simulink model "ACCLogic_Test_Template"  (R2022b)
settings: Solver=FixedStepAuto  StartTime=0.0  StopTime=35  RelTol=1e-3  EnableMultiTasking=on
InitFcn:
  | ACCLogic_TestCase1
StopFcn:
  | ACCLogic_Plot
values from neighbouring files (symbols this model uses):
  Car1_start_s = 140    [ACCLogic_TestCase1.m]    (also in ACCLogic_TestCase2.m = 30)
  Car1_us = 0    [ACCLogic_TestCase1.m]    (also in ACCLogic_TestCase2.m)
  Car2_start_s = 42    [ACCLogic_TestCase1.m]    (also in ACCLogic_TestCase2.m = 47)
  Car2_us = 1.25    [ACCLogic_TestCase1.m]    (also in ACCLogic_TestCase2.m = 1)
  Car3_start_s = 25    [ACCLogic_TestCase1.m]    (also in ACCLogic_TestCase2.m)
  Car3_us = 0.25    [ACCLogic_TestCase1.m]    (also in ACCLogic_TestCase2.m)
  Car4_start_s = 95    [ACCLogic_TestCase1.m]    (also in ACCLogic_TestCase2.m = 35)
  Car4_us = 0.5    [ACCLogic_TestCase1.m]    (also in ACCLogic_TestCase2.m)
  Car5_start_s = 141    [ACCLogic_TestCase1.m]    (also in ACCLogic_TestCase2.m = 75)
  Car5_us = 0    [ACCLogic_TestCase1.m]    (also in ACCLogic_TestCase2.m)
  Car6_start_s = 142    [ACCLogic_TestCase1.m]    (also in ACCLogic_TestCase2.m = 30)
  Car6_us = 0    [ACCLogic_TestCase1.m]    (also in ACCLogic_TestCase2.m = 0.2)
  ManEnt1 = 10    [ACCLogic_TestCase1.m]    (also in ACCLogic_TestCase2.m)
  ManEnt2 = 15    [ACCLogic_TestCase1.m]    (also in ACCLogic_TestCase2.m)
  ManEnt3 = 20    [ACCLogic_TestCase1.m]    (also in ACCLogic_TestCase2.m)
  ManEnt4 = 25    [ACCLogic_TestCase1.m]    (also in ACCLogic_TestCase2.m)
  MyCarMan_us = 6    [ACCLogic_TestCase1.m]    (also in ACCLogic_TestCase2.m)
  MyCarVel_us = 3    [ACCLogic_TestCase1.m]    (also in ACCLogic_TestCase2.m)
  TIMESTEP = 0.01    [ACCLogic_TestCase1.m]    (also in ACCLogic_TestCase2.m)
libraries: simulink x6
settings Model: Creator=raoulkumar  LastModifiedBy=ryshaw
settings SolverCC: AlgebraicLoopSolver=TrustRegion
settings DataIOCC: SaveFormat=Array  ReturnWorkspaceOutputs=off
settings OptimizationCC: LifeSpan=inf
settings DebuggingCC: UnconnectedInputMsg=warning  UnconnectedOutputMsg=warning  UnconnectedLineMsg=warning  AllowSymbolicDim=off  SFUnexpectedBacktrackingDiag=warning  SFNoUnconditionalDefaultTransitionDiag=warning  SFExecutionAtInitializationDiag=none  SFMachineParentedDataDiag=warning  ArithmeticOperatorsInVariantConditions=warning
settings ModelReferenceCC: EnableRefExpFcnMdlSchedulingChecks=on  PropagateSignalLabelsOutOfModel=off
settings SFSimCC: SimUseLocalCustomCode=off  CustomCodeUndefinedFunction=UseInterfaceOnly
settings RTWCC: RTWUseLocalCustomCode=off
settings CodeAppCC: StateflowObjectComments=on
settings GRTTargetCC: TargetLangStandard=C89/C90 (ANSI)
settings ConfigComp: CovMetricSettings=dw  CovSaveCumulativeToWorkspaceVar=on  CovSaveSingleToWorkspaceVar=on  CovExternalEMLEnable=off

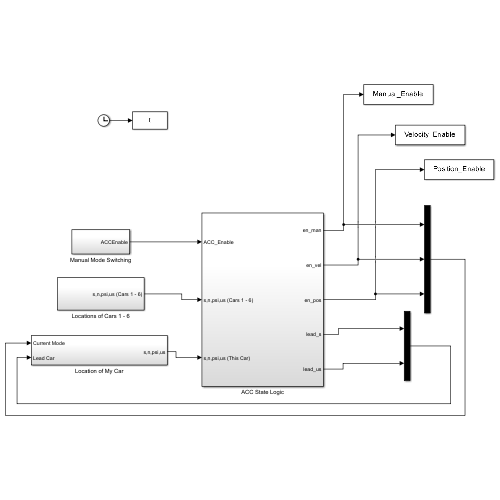
[thumbnail: Simulink's stored preview of the top-level diagram]
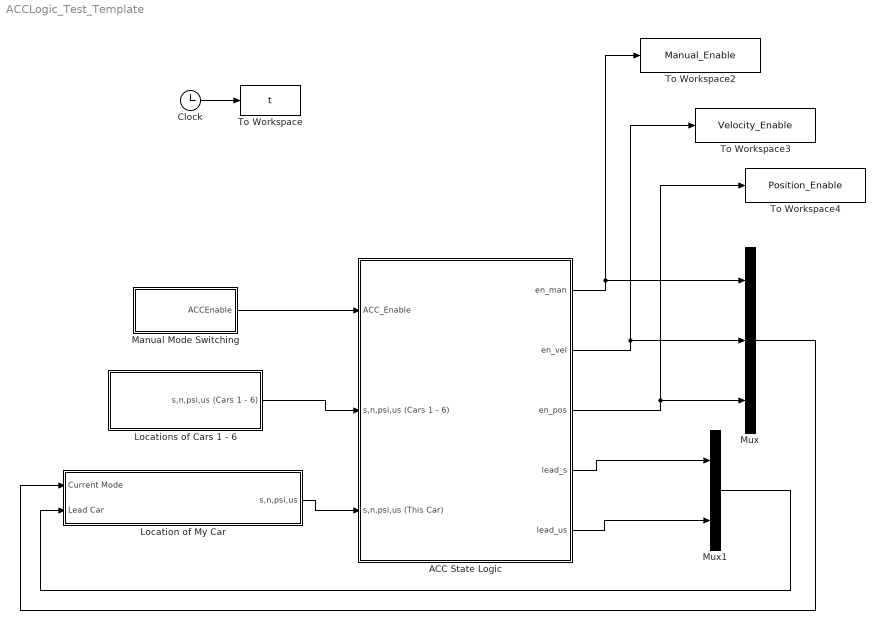
== system ACCLogic_Test_Template ==
  ACC State Logic : Subsystem
  Clock : Clock
  Location of My Car : Subsystem
  Locations of Cars 1 - 6 : Subsystem
  Manual Mode Switching : Subsystem
  Mux : Mux  Inputs=3
  Mux1 : Mux  Inputs=2
  To Workspace : ToWorkspace  VariableName=t  SampleTime=-1
  To Workspace2 : ToWorkspace  VariableName=Manual_Enable  SampleTime=-1
  To Workspace3 : ToWorkspace  VariableName=Velocity_Enable  SampleTime=-1
  To Workspace4 : ToWorkspace  VariableName=Position_Enable  SampleTime=-1
  wires:
  Clock/1 -> To Workspace/1
  Manual Mode Switching/1(ACCEnable) -> ACC State Logic/1(ACC_Enable)
  Locations of Cars 1 - 6/1(s,n,psi,us (Cars 1 - 6)) -> ACC State Logic/2(s,n,psi,us (Cars 1 - 6))
  Location of My Car/1(s,n,psi,us) -> ACC State Logic/3(s,n,psi,us (This Car))
  ACC State Logic/1(en_man) -> To Workspace2/1, Mux/1
  ACC State Logic/2(en_vel) -> To Workspace3/1, Mux/2
  ACC State Logic/3(en_pos) -> To Workspace4/1, Mux/3
  ACC State Logic/4(lead_s) -> Mux1/1
  ACC State Logic/5(lead_us) -> Mux1/2
  Mux/1 -> Location of My Car/1(Current Mode)
  Mux1/1 -> Location of My Car/2(Lead Car)

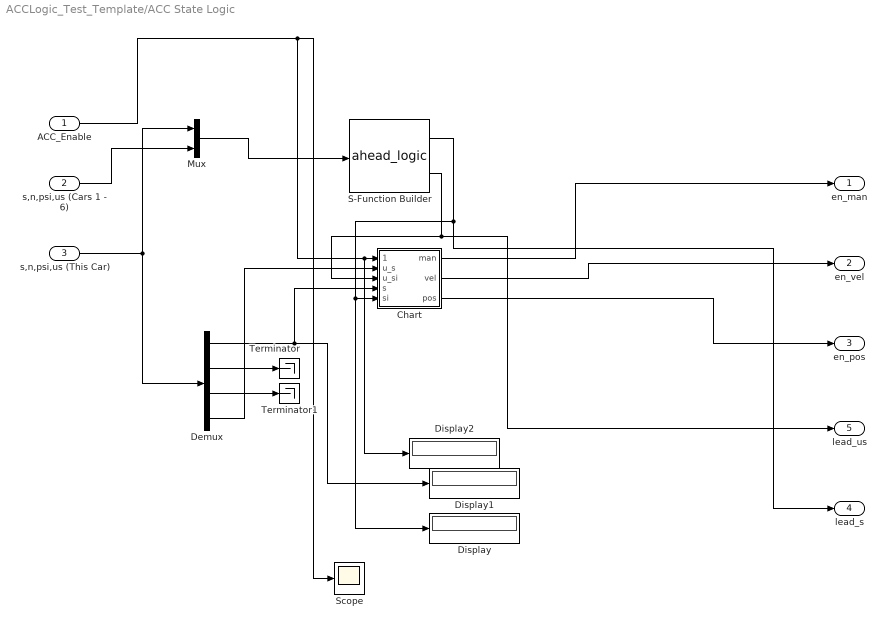
== system ACCLogic_Test_Template/ACC State Logic ==
  ACC_Enable : Inport
  s,n,psi,us (Cars 1 - 6) : Inport  Port=2
  s,n,psi,us (This Car) : Inport  Port=3
  Chart : Stateflow chart  TreatAsAtomicUnit=on
  Demux : Demux
  Display : Display
  Display1 : Display
  Display2 : Display
  Mux : Mux  Inputs=2
  S-Function Builder : S-Function  FunctionName=ahead_logic  SFunctionModules=ahead_logic_wrapper  SFunctionDeploymentMode=off  EnableBusSupport=off  mask(S-Function Builder){}
      mask help: Simulink:masks:SFunctionBuilder_MD
      mask init:
      | val = [[.9  0.75 0.75 1 1 .9 .9 1]',[1 1 0.75 0.75 .9 .9 1 .9]'];try , sys = get_param(gcb,'SfunBuilderFcnName');if isempty(sys), sys = get_param(gcb,'FunctionName'); end,catch, sys = get_param(gcb,'FunctionName'); end
      settings: CopyFcn=set_param(gcbh,'LinkStatus','none')  PreSaveFcn=try, set_param(gcb,'FunctionName','ahead_logic'), end  OpenFcn=sfunctionwizard(gcbh)
      mask Display: plot(val(:,1),val(:,2)),disp(sys), port_label('input',1,'u'), port_label('output',1,'s_out'), port_label('output',2,'us_out')
  Scope : Scope
  Terminator : Terminator
  Terminator1 : Terminator
  en_man : Outport
  en_vel : Outport  Port=2
  en_pos : Outport  Port=3
  lead_s : Outport  Port=4
  lead_us : Outport  Port=5
  wires:
  Chart/2(vel) -> en_vel/1
  Chart/1(man) -> en_man/1
  S-Function Builder/2 -> lead_us/1, Chart/3(u_si)
  Demux/2 -> Terminator/1
  Demux/1 -> Chart/4(s), Display1/1
  s,n,psi,us (Cars 1 - 6)/1 -> Mux/2
  Demux/3 -> Terminator1/1
  Mux/1 -> S-Function Builder/1
  Chart/3(pos) -> en_pos/1
  S-Function Builder/1 -> lead_s/1, Chart/5(si), Display/1
  Demux/4 -> Chart/2(u_s)
  s,n,psi,us (This Car)/1 -> Demux/1, Mux/1
  ACC_Enable/1 -> Scope/1, Chart/1(acc_en), Display2/1

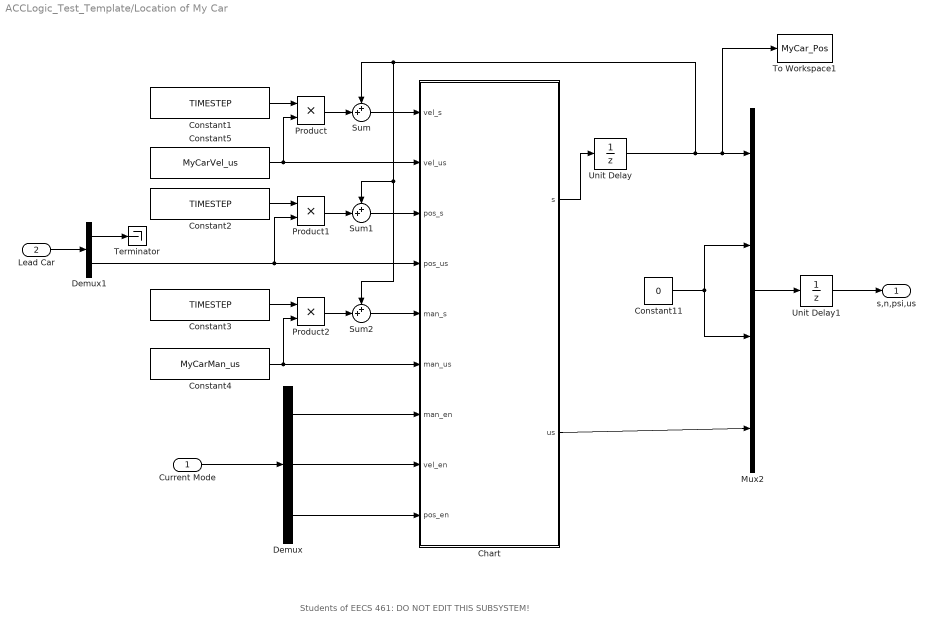
== system ACCLogic_Test_Template/Location of My Car ==
  note: Students of EECS 461: DO NOT EDIT THIS SUBSYSTEM!
  Current Mode : Inport
  Lead Car : Inport  Port=2
  Chart : Stateflow chart  TreatAsAtomicUnit=on
  Constant1 : Constant  Value=TIMESTEP  OutDataTypeStr=single
  Constant11 : Constant  Value=0  OutDataTypeStr=single
  Constant2 : Constant  Value=TIMESTEP  OutDataTypeStr=single
  Constant3 : Constant  Value=TIMESTEP  OutDataTypeStr=single
  Constant4 : Constant  Value=MyCarMan_us  OutDataTypeStr=single
  Constant5 : Constant  Value=MyCarVel_us  OutDataTypeStr=single
  Demux : Demux  Outputs=3
  Demux1 : Demux  Outputs=2
  Mux2 : Mux
  Product : Product  RndMeth=Zero
  Product1 : Product  RndMeth=Zero
  Product2 : Product  RndMeth=Zero
  Sum : Sum  Inputs=++|
  Sum1 : Sum  Inputs=++|
  Sum2 : Sum  Inputs=++|
  Terminator : Terminator
  To Workspace1 : ToWorkspace  VariableName=MyCar_Pos  SampleTime=-1
  Unit Delay : UnitDelay  SampleTime=TIMESTEP  HasFrameUpgradeWarning=on
  Unit Delay1 : UnitDelay  SampleTime=TIMESTEP  HasFrameUpgradeWarning=on
  s,n,psi,us : Outport
  wires:
  Chart/2(us) -> Mux2/4
  Demux/1 -> Chart/7(man_en)
  Demux/2 -> Chart/8(vel_en)
  Demux/3 -> Chart/9(pos_en)
  Sum/1 -> Chart/1(vel_s)
  Product/1 -> Sum/2
  Constant1/1 -> Product/1
  Product1/1 -> Sum1/2
  Constant2/1 -> Product1/1
  Sum1/1 -> Chart/3(pos_s)
  Sum2/1 -> Chart/5(man_s)
  Product2/1 -> Sum2/2
  Constant3/1 -> Product2/1
  Chart/1(s) -> Unit Delay/1
  Unit Delay/1 -> Mux2/1, To Workspace1/1, Sum/1, Sum1/1, Sum2/1
  Mux2/1 -> Unit Delay1/1
  Unit Delay1/1 -> s,n,psi,us/1
  Current Mode/1 -> Demux/1
  Constant4/1 -> Chart/6(man_us), Product2/2
  Constant5/1 -> Chart/2(vel_us), Product/2
  Constant11/1 -> Mux2/2, Mux2/3
  Lead Car/1 -> Demux1/1
  Demux1/1 -> Terminator/1
  Demux1/2 -> Chart/4(pos_us), Product1/2

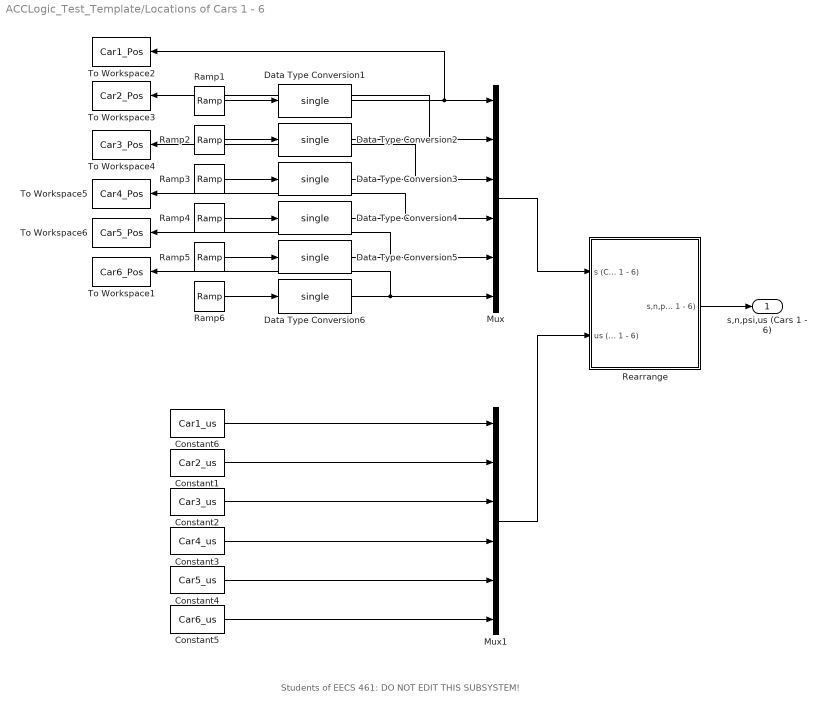
== system ACCLogic_Test_Template/Locations of Cars 1 - 6 ==
  note: Students of EECS 461: DO NOT EDIT THIS SUBSYSTEM!
  Constant1 : Constant  Value=Car2_us  OutDataTypeStr=single
  Constant2 : Constant  Value=Car3_us  OutDataTypeStr=single
  Constant3 : Constant  Value=Car4_us  OutDataTypeStr=single
  Constant4 : Constant  Value=Car5_us  OutDataTypeStr=single
  Constant5 : Constant  Value=Car6_us  OutDataTypeStr=single
  Constant6 : Constant  Value=Car1_us  OutDataTypeStr=single
  Data Type Conversion{1..6} (6 alike) : DataTypeConversion  OutDataTypeStr=single  SaturateOnIntegerOverflow=off  RndMeth=Floor
  Mux : Mux  Inputs=6
  Mux1 : Mux  Inputs=6
  Ramp1 : simulink/Sources/Ramp  slope=Car1_us  start=0  InitialOutput=Car1_start_s
  Ramp2 : simulink/Sources/Ramp  slope=Car2_us  start=0  InitialOutput=Car2_start_s
  Ramp3 : simulink/Sources/Ramp  slope=Car3_us  start=0  InitialOutput=Car3_start_s
  Ramp4 : simulink/Sources/Ramp  slope=Car4_us  start=0  InitialOutput=Car4_start_s
  Ramp5 : simulink/Sources/Ramp  slope=Car5_us  start=0  InitialOutput=Car5_start_s
  Ramp6 : simulink/Sources/Ramp  slope=Car6_us  start=0  InitialOutput=Car6_start_s
  Rearrange : Subsystem
  To Workspace1 : ToWorkspace  VariableName=Car6_Pos  SampleTime=-1
  To Workspace2 : ToWorkspace  VariableName=Car1_Pos  SampleTime=-1
  To Workspace3 : ToWorkspace  VariableName=Car2_Pos  SampleTime=-1
  To Workspace4 : ToWorkspace  VariableName=Car3_Pos  SampleTime=-1
  To Workspace5 : ToWorkspace  VariableName=Car4_Pos  SampleTime=-1
  To Workspace6 : ToWorkspace  VariableName=Car5_Pos  SampleTime=-1
  s,n,psi,us (Cars 1 - 6) : Outport
  wires:
  Constant6/1 -> Mux1/1
  Constant1/1 -> Mux1/2
  Constant2/1 -> Mux1/3
  Constant3/1 -> Mux1/4
  Constant4/1 -> Mux1/5
  Mux/1 -> Rearrange/1(s (Cars 1 - 6))
  Mux1/1 -> Rearrange/2(us (Cars 1 - 6))
  Ramp1/1 -> Data Type Conversion1/1
  Data Type Conversion1/1 -> Mux/1, To Workspace2/1
  Ramp2/1 -> Data Type Conversion2/1
  Data Type Conversion2/1 -> To Workspace3/1, Mux/2
  Ramp3/1 -> Data Type Conversion3/1
  Data Type Conversion3/1 -> Mux/3, To Workspace4/1
  Ramp4/1 -> Data Type Conversion4/1
  Data Type Conversion4/1 -> Mux/4, To Workspace5/1
  Ramp5/1 -> Data Type Conversion5/1
  Data Type Conversion5/1 -> Mux/5, To Workspace6/1
  Rearrange/1(s,n,psi,us (Cars 1 - 6)) -> s,n,psi,us (Cars 1 - 6)/1
  Ramp6/1 -> Data Type Conversion6/1
  Data Type Conversion6/1 -> Mux/6, To Workspace1/1
  Constant5/1 -> Mux1/6

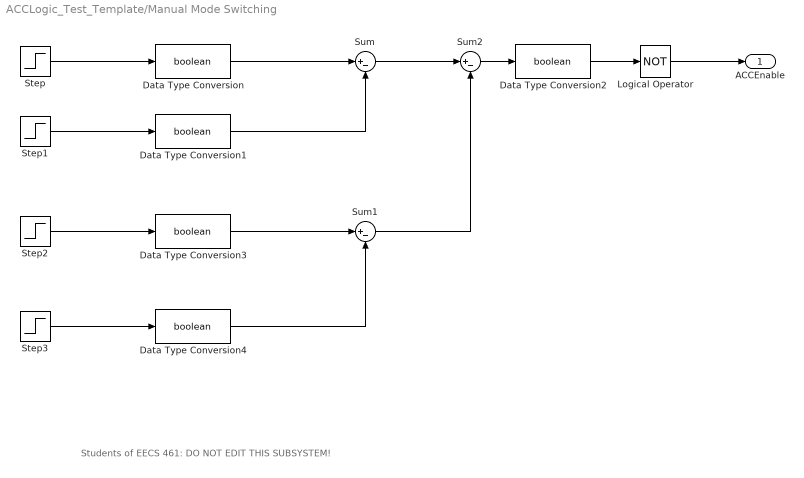
== system ACCLogic_Test_Template/Manual Mode Switching ==
  note: Students of EECS 461: DO NOT EDIT THIS SUBSYSTEM!
  Data Type Conversion{,1..4} (5 alike) : DataTypeConversion  OutDataTypeStr=boolean  SaturateOnIntegerOverflow=off  RndMeth=Floor
  Logical Operator : Logic  Operator=NOT  AllPortsSameDT=off  OutDataTypeStr=boolean
  Step : Step  Time=ManEnt1  SampleTime=0
  Step1 : Step  Time=ManEnt2  SampleTime=0
  Step2 : Step  Time=ManEnt3  SampleTime=0
  Step3 : Step  Time=ManEnt4  SampleTime=0
  Sum : Sum  Inputs=|+-
  Sum1 : Sum  Inputs=|+-
  Sum2 : Sum  Inputs=|+-
  ACCEnable : Outport
  wires:
  Step/1 -> Data Type Conversion/1
  Step1/1 -> Data Type Conversion1/1
  Data Type Conversion/1 -> Sum/1
  Data Type Conversion1/1 -> Sum/2
  Data Type Conversion2/1 -> Logical Operator/1
  Step2/1 -> Data Type Conversion3/1
  Step3/1 -> Data Type Conversion4/1
  Data Type Conversion3/1 -> Sum1/1
  Data Type Conversion4/1 -> Sum1/2
  Sum/1 -> Sum2/1
  Sum1/1 -> Sum2/2
  Sum2/1 -> Data Type Conversion2/1
  Logical Operator/1 -> ACCEnable/1

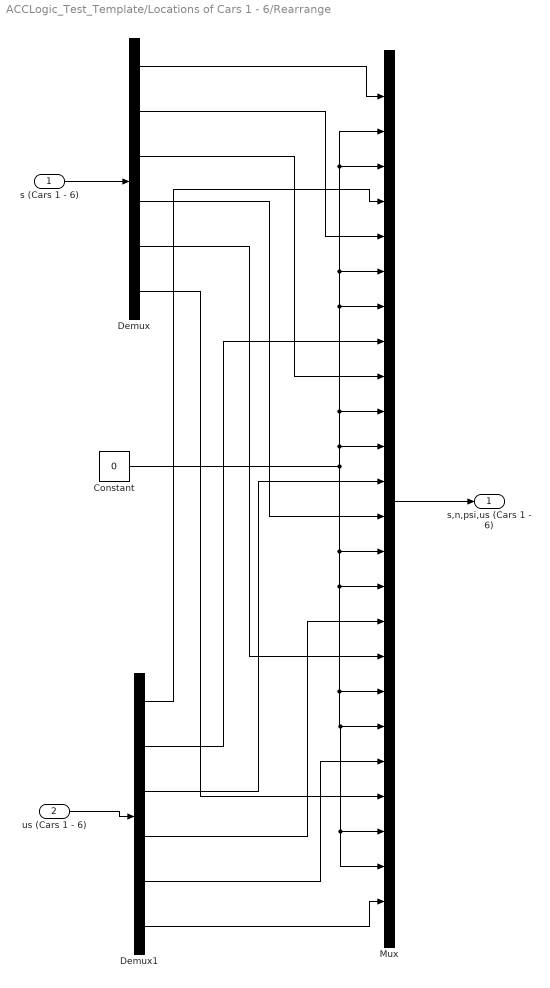
== system ACCLogic_Test_Template/Locations of Cars 1 - 6/Rearrange ==
  s (Cars 1 - 6) : Inport
  us (Cars 1 - 6) : Inport  Port=2
  Constant : Constant  Value=0  OutDataTypeStr=single
  Demux : Demux  Outputs=6
  Demux1 : Demux  Outputs=6
  Mux : Mux  Inputs=24
  s,n,psi,us (Cars 1 - 6) : Outport
  wires:
  us (Cars 1 - 6)/1 -> Demux1/1
  s (Cars 1 - 6)/1 -> Demux/1
  Demux/1 -> Mux/1
  Constant/1 -> Mux/18, Mux/23, Mux/22, Mux/19, Mux/15, Mux/14, Mux/11, Mux/2, Mux/3, Mux/6, Mux/7, Mux/10
  Demux1/1 -> Mux/4
  Demux/2 -> Mux/5
  Demux1/2 -> Mux/8
  Demux/3 -> Mux/9
  Demux1/3 -> Mux/12
  Demux/4 -> Mux/13
  Demux1/4 -> Mux/16
  Demux/5 -> Mux/17
  Demux1/5 -> Mux/20
  Mux/1 -> s,n,psi,us (Cars 1 - 6)/1
  Demux1/6 -> Mux/24
  Demux/6 -> Mux/21

== stateflow chart ACCLogic_Test_Template/Location of My Car/Chart ==
  state vel_ctrl
    during:s = vel_s
    during:us = vel_us
  state pos_ctrl
    during:s = pos_s
    during:us = pos_us
  state man_ctrl
    during:s = man_s
    during:us = man_us
  (default) -> vel_ctrl
  vel_ctrl -> pos_ctrl [order 1] : [(pos_en==1)&(vel_en==0)&(man_en==0)]
  pos_ctrl -> vel_ctrl [order 1] : [(pos_en == 0)&(vel_en == 1)&(man_en == 0)]
  vel_ctrl -> man_ctrl [order 2] : [(pos_en == 0)&(vel_en == 0)&(man_en == 1)]
  man_ctrl -> vel_ctrl [order 2] : [(pos_en == 0)&(vel_en == 1)&(man_en == 0)]
  pos_ctrl -> man_ctrl [order 2] : [(pos_en == 0)&(vel_en == 0)&(man_en == 1)]
  man_ctrl -> pos_ctrl [order 1] : [(pos_en == 1)&(vel_en == 0)&(man_en == 0)]
  data: vel_s input single; vel_us input single; pos_s input single; pos_us input single; man_s input single; man_us input single; man_en input boolean; vel_en input boolean; pos_en input boolean; s output single; us output single

== stateflow chart ACCLogic_Test_Template/ACC State Logic/Chart ==
  state Manual
    during:
    man = true;
    vel = false;
    pos = false;
  state PosCtrl
    during:
    man = false;
    vel = false;
    pos = true;
  state VelCtrl
    during:
    man = false;
    vel = true;
    pos = false;
  (default) -> Manual
  Manual -> PosCtrl [order 1] : [acc_en && (u_si <= u_s && (si - s) <= H && (u_si ~= u_s))]
  PosCtrl -> Manual [order 1] : [~acc_en]
  VelCtrl -> Manual [order 1] : [~acc_en]
  Manual -> VelCtrl [order 2] : [acc_en && (u_si > u_s || (si - s) > H || (u_si == u_s))]
  PosCtrl -> VelCtrl [order 2] : [acc_en && (u_si > u_s || (si - s) > H  || (u_si == u_s)) && u_si - u_s > 1]
  VelCtrl -> PosCtrl [order 2] : [acc_en && (u_si <= u_s && (si - s) <= H && (u_si ~= u_s))]
  data: acc_en input; man output boolean; vel output boolean; H parameter; pos output boolean; u_s input; u_si input; s input; si input
